simulink model "model_for_testing_errors"  (R2023b)
settings: Solver=VariableStepAuto  StartTime=0.0  StopTime=time_model  FixedStep=0.0001  RelTol=1e-3
values from neighbouring files (symbols this model uses):
  A_flap = [c_a, c_b, 0 ... (first row only)    [LQR_calculate.m]    (also in LQR_feedback.m; LQR_linearized_test.m; MPC_test.m; MPC_test_1.m)
  A_ind = [c_d, 0, 0 ... (first row only)    [LQR_calculate.m]    (also in LQR_feedback.m; LQR_linearized_test.m; MPC_test.m; MPC_test_1.m)
  C_drag = 0    [LQR_calculate.m]    (also in LQR_feedback.m = C_drag_arr(i); LQR_linearized_test.m = C_drag_arr(i); MPC_test.m = C_drag_arr(i); MPC_test_1.m = C_drag_arr(i))
  demp = 0    [LQR_feedback.m]    (also in LQR_linearized_test.m; MPC_params.m; MPC_test_1.m; initQuadrotorData.m)
  forward_1 = 20    [LQR_feedback.m]    (also in LQR_linearized_test.m; MPC_test_1.m)
  forward_2 = 20    [LQR_feedback.m]    (also in LQR_linearized_test.m; MPC_test_1.m)
  g = 9.81    [LQR_calculate.m]    (also in LQR_feedback.m = 9.8; LQR_linearized_test.m = 9.8; LQR_testing_gpt.m; MPC_params.m = 9.8)
  Im = 0.0135^2*0.045/2    (= 4.100625e-06)    [LQR_calculate.m]    (also in LQR_feedback.m; LQR_linearized_test.m; MPC_params.m; MPC_test.m)
  Ix = m/3*a^2/12+2*0.045*l^2    (= 0.00211347222222)    [LQR_calculate.m]    (also in LQR_feedback.m; LQR_linearized_test.m; LQR_testing_gpt.m = 0.0081; MPC_params.m)
  Iy = m/3*a^2/12+4*0.045*l^2    (= 0.00413847222222)    [LQR_calculate.m]    (also in LQR_feedback.m = 0.00211347222222; LQR_linearized_test.m = 0.00211347222222; LQR_testing_gpt.m = 0.0081; MPC_params.m = 0.00211347222222)
  Iz = m/3*a^2/4+2*0.045*l^2    (= 0.00229041666667)    [LQR_calculate.m]    (also in LQR_feedback.m = 0.00431541666667; LQR_linearized_test.m = 0.00431541666667; LQR_testing_gpt.m = 0.0142; MPC_params.m = 0.00431541666667)
  J = 2.5*10^(-6)    (= 2.5e-06)    [LQR_calculate.m]    (also in LQR_feedback.m; LQR_linearized_test.m; MPC_params.m; MPC_test.m)
  K = Y * inv(P)    [LQR_calculate.m]    (also in LQR_feedback.m = [Kx;Ky;Kz;Kphi;Ktheta;-Kpsi])
  Ke = ke    (= 0.0073)    [LQR_calculate.m]    (also in LQR_feedback.m = 0.00734; LQR_linearized_test.m = 0.00734; MPC_params.m = 0.00734; MPC_test.m)
  kf = ks*r^2*airDensity*Sblade/2    (= 1.57565625e-05)    [LQR_calculate.m]    (also in LQR_feedback.m; LQR_linearized_test.m; MPC_params.m; MPC_test.m)
  Km = kt    (= 0.0073)    [LQR_calculate.m]    (also in LQR_feedback.m = 0.00734; LQR_linearized_test.m = 0.00734; MPC_params.m = 0.00734; MPC_test.m)
  kv = 1300    [LQR_feedback.m]    (also in LQR_linearized_test.m; MPC_test_1.m; initQuadrotorData.m)
  l = 0.15    [LQR_calculate.m]    (also in LQR_feedback.m; LQR_linearized_test.m; MPC_params.m; MPC_test.m)
  L = La    (= 5e-05)    [LQR_calculate.m]    (also in LQR_feedback.m = 0.0001; LQR_linearized_test.m = 0.0001; MPC_params.m = 0.0001; MPC_test.m)
  m = size(B, 2)    [LQR_calculate.m]    (also in LQR_feedback.m = 0.65; LQR_linearized_test.m = 0.65; LQR_testing_gpt.m = 1; MPC_params.m = 0.65)
  Mode = 3    [LQR_feedback.m]    (also in LQR_linearized_test.m; MPC_test_1.m = 1)
  phi0 = 0    [LQR_feedback.m]    (also in LQR_linearized_test.m; MPC_test_1.m)
  psi0 = pi/2    (= 1.57079632679)    [LQR_feedback.m]    (also in LQR_linearized_test.m; MPC_test_1.m = 0)
  Psid = 0    [LQR_feedback.m]    (also in LQR_linearized_test.m; MPC_test_1.m)
  R = eye(4)    [LQR_calculate.m]    (also in LQR_feedback.m = 0.058; LQR_linearized_test.m = 0.058; LQR_testing_gpt.m = diag([0.1, 10, 100, 10]); MPC_params.m = 0.058)
  rho = 1.225    [LQR_calculate.m]    (also in LQR_feedback.m; LQR_linearized_test.m; MPC_params.m; MPC_test.m)
  S = l*c*4+a*b    (= 0.0169)    [LQR_calculate.m]    (also in LQR_feedback.m; LQR_linearized_test.m; MPC_params.m; MPC_test.m)
  theta0 = 0    [LQR_feedback.m]    (also in LQR_linearized_test.m; MPC_test_1.m)
  time_model = time_model_arr(i)    [LQR_feedback.m]    (also in LQR_linearized_test.m; MPC_test.m; MPC_test_1.m; plot_model_out.m)
  total_time = 60    [LQR_feedback.m]    (also in LQR_linearized_test.m; MPC_test_1.m)
  up_down = 5    [LQR_feedback.m]    (also in LQR_linearized_test.m; MPC_test_1.m)
  x0 = 0    [LQR_feedback.m]    (also in LQR_linearized_test.m; MPC_test_1.m; init_nmpc.m = zeros(nx,1))
  Xd = [Simulation.trajectory.Data(1,:)',Simulation.trajectory.Data(2,:)',Simulation.trajectory.Data(3,:)',Simulation.trajectory.Data(9,:)']    [LQR_feedback.m]    (also in LQR_linearized_test.m; MPC_test_1.m; plot_model_out.m)
  y0 = 0    [LQR_feedback.m]    (also in LQR_linearized_test.m; MPC_test_1.m)
  Yd = 0    [LQR_feedback.m]    (also in LQR_linearized_test.m; MPC_test_1.m)
  z0 = 0    [LQR_feedback.m]    (also in LQR_linearized_test.m; MPC_test_1.m)
  Zd = 0    [LQR_feedback.m]    (also in LQR_linearized_test.m; MPC_test_1.m)
libraries: sharedtransform x1
(part 2 of 2)

== matlab function model_for_testing_errors/MATLAB Function ==
  data: t input; forward_20 input; x_ref output; forward_10 input; up_down input; total_time input
function x_ref = generate_quadcopter_route_real_time(t, forward_20, forward_10, up_down, total_time)
    % Доля времени на повороты
    turn_time_ratio = 0.2;
    total_turn_time = total_time * turn_time_ratio;
    total_linear_time = total_time - total_turn_time;

    % Время на каждый поворот
    turn_time = total_turn_time / 4;

    % Линейные сегменты разбиты на движение по XY и по Z (всего 8 отрезков)
    % Формат: [dx, dy, dz, dpsi]
    segments = [
        forward_20, 0, 0, 0;       % вперед
        0, 0, up_down, 0;          % вверх
        0, 0, 0, -pi/2;             % поворот влево
        forward_10, 0, 0, 0;       % вперед
        0, 0, -up_down, 0;         % вниз
        0, 0, 0, -pi/2;             % поворот влево
        forward_20, 0, 0, 0;       % вперед
        0, 0, up_down, 0;          % вверх
        0, 0, 0, -pi/2;             % поворот влево
        forward_10, 0, 0, 0;       % вперед
        0, 0, -up_down, 0;         % вниз
        0, 0, 0, -pi/2;             % поворот влево
    ];

    % Определяем длину каждого линейного сегмента
    segment_lengths = vecnorm(segments(:, 1:3), 2, 2);
    total_path_length = sum(segment_lengths);
    
    % Распределяем время на каждый линейный сегмент пропорционально длине
    segment_times = zeros(size(segments, 1), 1);
    for i = 1:size(segments, 1)
        if segments(i, 4) == 0 % линейное движение
            segment_times(i) = segment_lengths(i) / total_path_length * total_linear_time;
        else % поворот
            segment_times(i) = turn_time;
        end
    end

    % Инициализация
    current_x = 0;
    current_y = 0;
    current_z = 0;
    current_psi = 0;
    accumulated_time = 0;

    % Обход сегментов
    for s = 1:size(segments, 1)
        dt = segment_times(s);
        if t <= accumulated_time + dt || s == size(segments,1)
            % Текущий сегмент
            segment_progress = (t - accumulated_time) / dt;
            segment_progress = max(0, min(1, segment_progress));

            dx = segments(s, 1) * segment_progress;
            dy = segments(s, 2) * segment_progress;
            dz = segments(s, 3) * segment_progress;
            dpsi = segments(s, 4) * segment_progress;

            % Преобразование координат с учетом текущего поворота
            if dx ~= 0 || dy ~= 0
                R = [cos(current_psi), -sin(current_psi);
                     sin(current_psi),  cos(current_psi)];
                xy = R * [dx; dy];
            else
                xy = [0; 0];
            end

            x = current_x + xy(1);
            y = current_y + xy(2);
            z = current_z + dz;
            psi = current_psi + dpsi;

            x_ref = [x; y; z; 0; 0; 0; 0; 0; psi; 0; 0; 0];
            return;
        end

        % Завершённый сегмент — обновляем позицию
        dx = segments(s, 1);
        dy = segments(s, 2);
        dz = segments(s, 3);
        dpsi = segments(s, 4);

        if dx ~= 0 || dy ~= 0
            R = [cos(current_psi), -sin(current_psi);
                 sin(current_psi),  cos(current_psi)];
            xy = R * [dx; dy];
        else
            xy = [0; 0];
        end

        current_x = current_x + xy(1);
        current_y = current_y + xy(2);
        current_z = current_z + dz;
        current_psi = current_psi + dpsi;

        accumulated_time = accumulated_time + segment_times(s);
    end

    % Если всё завершено — остаёмся в конечной точке
    x_ref = [current_x; current_y; current_z; 0; 0; 0; 0; 0; current_psi; 0; 0; 0];
end

== matlab function model_for_testing_errors/MATLAB Function1 ==
  data: t input; x_ref output
function x_ref = trajectory_generator(t)
%#codegen

% Параметры восьмерки
A = 10;      % амплитуда по x
B = 6.5;    % амплитуда по y
h = 5;      % высота
w = 0.5;    % частота

% Параметризация
x = A * sin(w * t);
y = B * sin(w * t) * cos(w * t);
z = h;

% Вычислим производные для курса
dx = A * w * cos(w * t);
dy = B * w * cos(2 * w * t);

% Курс (ориентация по траектории)
psi = atan2(dy, dx);  % направление движенияs

% Выход
x_ref = [x; y; z; 0;0;0;0;0; psi;0;0;0];
end

== matlab function model_for_testing_errors/Quadrotor System/Gyroscope ==
  data: w_1 input; w_2 input; w_3 input; w_Gamma output; w_4 input
function w_Gamma = fcn(w_1, w_2, w_3, w_4)
    
w_Gamma = w_1 - w_2 + w_3 - w_4;

== matlab function model_for_testing_errors/MATLAB Function2 ==
  data: X input; Y input; Z input; psi input; t input; x_ref output; time_model input; x0 input; y0 input; z0 input; psi0 input
function x_ref = linearTrajectory(X, Y, Z, psi, t, time_model, x0, y0, z0, psi0)
%#codegen
% Линейная интерполяция между начальной и конечной точками

% Инициализация прогресса
if time_model <= 0
    progress = 1.0;
else
    progress = min(t / time_model, 1.0);
end

% Расчет текущих координат
x_out = x0 + (X - x0) * progress;
y_out = y0 + (Y - y0) * progress;
z_out = z0 + (Z - z0) * progress;

% Расчет текущего угла (линейная интерполяция угла)
psi_out = psi0 + (psi - psi0) * progress;

x_ref = [x_out; y_out; z_out; 0;0;0;0;0; psi_out;0;0;0];
end
